simulink model "Tut18_BusAndMux"  (R2021a)
settings: Solver=VariableStepAuto  StartTime=0.0  StopTime=10.0  RelTol=1e-3
settings Model: Creator=cheta  LastModifiedBy=cheta

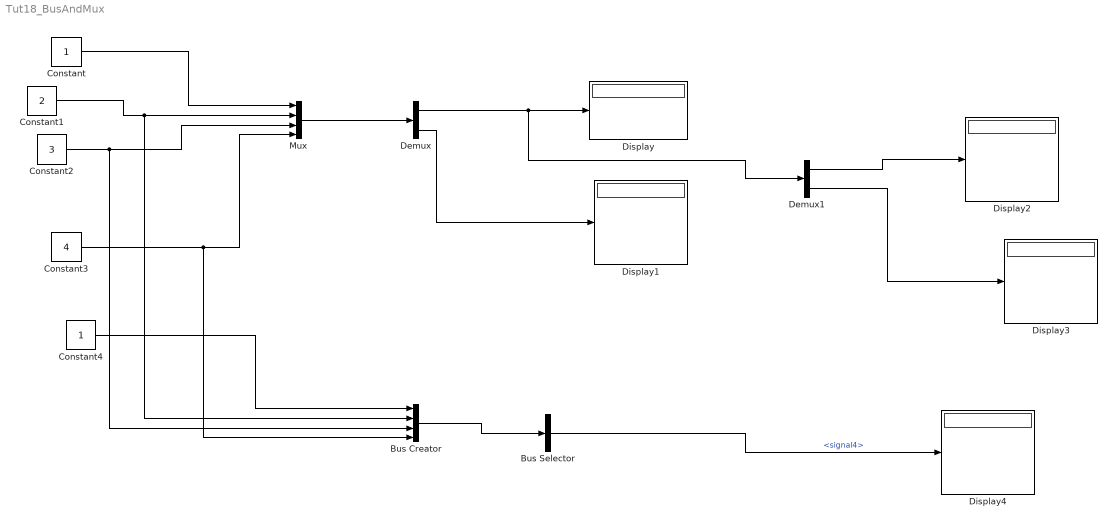
== system Tut18_BusAndMux ==
  Bus Creator : BusCreator  Inputs=4
  Bus Selector : BusSelector  OutputSignals=signal4
  Constant : Constant
  Constant1 : Constant  Value=2
  Constant2 : Constant  Value=3
  Constant3 : Constant  Value=4
  Constant4 : Constant  OutDataTypeStr=boolean
  Demux : Demux  Outputs=2
  Demux1 : Demux  Outputs=2
  Display{,1..4} (5 alike) : Display
  Mux : Mux
  wires:
  Constant/1 -> Mux/1
  Constant1/1 -> Bus Creator/2, Mux/2
  Constant2/1 -> Bus Creator/3, Mux/3
  Constant3/1 -> Bus Creator/4, Mux/4
  Mux/1 -> Demux/1
  Demux/1 -> Demux1/1, Display/1
  Demux/2 -> Display1/1
  Demux1/1 -> Display2/1
  Demux1/2 -> Display3/1
  Constant4/1 -> Bus Creator/1
  Bus Creator/1 -> Bus Selector/1
  Bus Selector/1 -> Display4/1  "<signal4>"
